simulink model "Battery_detailed_SOC_estimation"  (R2023b)
settings: Solver=VariableStepAuto  StartTime=0.0  StopTime=6*3600  RelTol=1e-3
InitFcn:
  | initialSOC = 0.5;
  | Ts = 1;
libraries: nesl_utility x4, fl_lib x3, simulink x3, batteryecm_lib x1
settings Model: Creator=arvba41  LastModifiedBy=arvba41

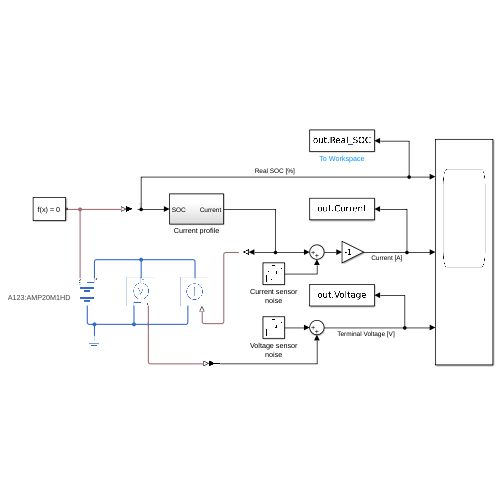
[thumbnail: Simulink's stored preview of the top-level diagram]
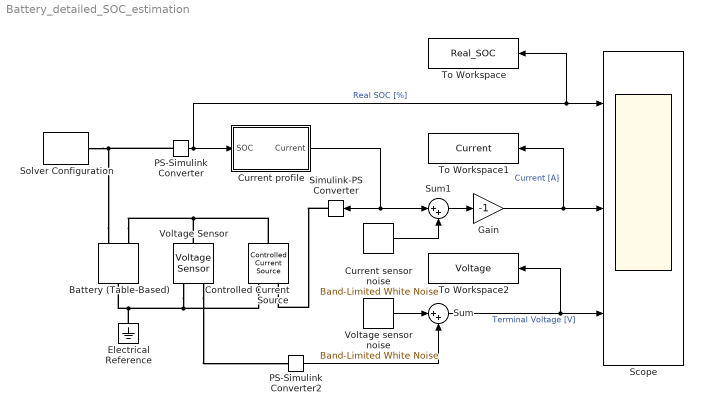
== system Battery_detailed_SOC_estimation ==
  Battery (Table-Based) : batteryecm_lib/Battery (Table-Based)  Tag={'toolbox/physmod/battery/shared_library/m/batteryecm_lib_parts';'Battery__Table_Based_/A123/AMP20M1HD.xml'}  SOC_vec=[0 0.01 0.02 0.03 0.04 0.05 0.06 0.07 0.08 0.09 0.1 0.11 0.12 0.13 0.14 0.15 0.16 0.17 0.18 0.19 0.2 0.21 0.22 0.23 0.24 0.25 0.26 0.27 0.28 0.29 0.3 0.31 0.32 0.33 0.34 0.35 0.36 0.37 0.38 0.39 0.4 0.41 0.42 0.43 0.44 0.45 0.46 0.47 0.48 0.49 0.5 0.51 0.52 0.53 0.54 0.55 0.56 0.57 0.58 0.59 0.6 0.61 0.62 0.63 0.64 0.65 0.66 0.67 0.68 0.69 0.7 0.71 0.72 0.73 0.74 0.75 0.76 0.77 0.78 0.79 0.8 0.81 0.82 0.83 0.84 0.85 0.86 0.87 0.88 0.89 0.9 0.91 0.92 0.93 0.94 0.95 0.96 0.97 0.98 0.99 1]  T_dependence=simscape.enum.tablebattery.temperature_dependence.yes  prm_dir=simscape.enum.tablebattery.prm_dir.noCurrentDirectionality  T_vec=[-10 0 10 25 35] degC  V0_mat=[2.93217 2.93217 2.93217 2.93217 2.93217;2.94263 2.94263 2.94263 2.94263 2.94263;2.95309 2.95309 2.95309 2.95309 2.95309;2.96355 2.96355 2.96355 2.96355 2.96355;2.97401 2.97401 2.97401 2.97401 2.97401;2.98447 2.98447 2.98447 2.98447 2.98447;2.99493 2.99493 2.99493 2.99493 2.99493;3.02455 3.02455 3.02455 3.02455 3.02455;3.05382 3.05382 3.05382 3.05382 3.05382;3.07377 3.07377 3.07377 3.07377 3.07377;3.08453 3.08453 3.08453 3.08453 3.08453;3.09529 3.09529 3.09529 3.09529 3.09529;3.09916 3.09916 3.09916 3.09916 3.09916;3.10271 3.10271 3.10271 3.10271 3.10271;3.10625 3.10625 3.10625 3.10625 3.10625;3.1098 3.1098 3.1098 3.1098 3.1098;3.11335 3.11335 3.11335 3.11335 3.11335;3.11689 3.11689 3.11689 3.11689 3.11689;3.12044 3.12044 3.12044 3.12044 3.12044;3.13089 3.13089 3.13089 3.13089 3.13089;3.13795 3.13795 3.13795 3.13795 3.13795;3.14459 3.14459 3.14459 3.14459 3.14459;3.14961 3.14961 3.14961 3.14961 3.14961;3.15451 3.15451 3.15451 3.15451 3.15451;3.15932 3.15932 3.15932 3.15932 3.15932;3.16324 3.16324 3.16324 3.16324 3.16324;3.16716 3.16716 3.16716 3.16716 3.16716;3.17063 3.17063 3.17063 3.17063 3.17063;3.17297 3.17297 3.17297 3.17297 3.17297;3.17544 3.17544 3.17544 3.17544 3.17544;3.17798 3.17798 3.17798 3.17798 3.17798;3.18052 3.18052 3.18052 3.18052 3.18052;3.18295 3.18295 3.18295 3.18295 3.18295;3.18533 3.18533 3.18533 3.18533 3.18533;3.18771 3.18771 3.18771 3.18771 3.18771;3.19009 3.19009 3.19009 3.19009 3.19009;3.19215 3.19215 3.19215 3.19215 3.19215;3.19403 3.19403 3.19403 3.19403 3.19403;3.1959 3.1959 3.1959 3.1959 3.1959;3.19777 3.19777 3.19777 3.19777 3.19777;3.1998 3.1998 3.1998 3.1998 3.1998;3.20198 3.20198 3.20198 3.20198 3.20198;3.20371 3.20371 3.20371 3.20371 3.20371;3.20501 3.20501 3.20501 3.20501 3.20501;3.20619 3.20619 3.20619 3.20619 3.20619;3.20738 3.20738 3.20738 3.20738 3.20738;3.20856 3.20856 3.20856 3.20856 3.20856;3.20974 3.20974 3.20974 3.20974 3.20974;3.21092 3.21092 3.21092 3.21092 3.21092;3.2121 3.2121 3.2121 3.2121 3.2121;3.21329 3.21329 3.21329 3.21329 3.21329;3.21447 3.21447 3.21447 3.21447 3.21447;3.21565 3.21565 3.21565 3.21565 3.21565;3.21672 3.21672 3.21672 3.21672 3.21672;3.21787 3.21787 3.21787 3.21787 3.21787;3.21904 3.21904 3.21904 3.21904 3.21904;3.22021 3.22021 3.22021 3.22021 3.22021;3.22139 3.22139 3.22139 3.22139 3.22139;3.22256 3.22256 3.22256 3.22256 3.22256;3.22374 3.22374 3.22374 3.22374 3.22374;3.22492 3.22492 3.22492 3.22492 3.22492;3.2261 3.2261 3.2261 3.2261 3.2261;3.22728 3.22728 3.22728 3.22728 3.22728;3.22847 3.22847 3.22847 3.22847 3.22847;3.22965 3.22965 3.22965 3.22965 3.22965;3.23083 3.23083 3.23083 3.23083 3.23083;3.23201 3.23201 3.23201 3.23201 3.23201;3.23319 3.23319 3.23319 3.23319 3.23319;3.23437 3.23437 3.23437 3.23437 3.23437;3.23552 3.23552 3.23552 3.23552 3.23552;3.23652 3.23652 3.23652 3.23652 3.23652;3.23778 3.23778 3.23778 3.23778 3.23778;3.23909 3.23909 3.23909 3.23909 3.23909;3.24045 3.24045 3.24045 3.24045 3.24045;3.24217 3.24217 3.24217 3.24217 3.24217;3.2439 3.2439 3.2439 3.2439 3.2439;3.24563 3.24563 3.24563 3.24563 3.24563;3.24736 3.24736 3.24736 3.24736 3.24736;3.24909 3.24909 3.24909 3.24909 3.24909;3.25082 3.25082 3.25082 3.25082 3.25082;3.25255 3.25255 3.25255 3.25255 3.25255;3.25428 3.25428 3.25428 3.25428 3.25428;3.256 3.256 3.256 3.256 3.256;3.25774 3.25774 3.25774 3.25774 3.25774;3.25951 3.25951 3.25951 3.25951 3.25951;3.26116 3.26116 3.26116 3.26116 3.26116;3.26238 3.26238 3.26238 3.26238 3.26238;3.26307 3.26307 3.26307 3.26307 3.26307;3.26352 3.26352 3.26352 3.26352 3.26352;3.26396 3.26396 3.26396 3.26396 3.26396;3.26441 3.26441 3.26441 3.26441 3.26441;3.26485 3.26485 3.26485 3.26485 3.26485;3.2653 3.2653 3.2653 3.2653 3.2653;3.26593 3.26593 3.26593 3.26593 3.26593;3.26612 3.26612 3.26612 3.26612 3.26612;3.26743 3.26743 3.26743 3.26743 3.26743;3.26879 3.26879 3.26879 3.26879 3.26879;3.27596 3.27596 3.27596 3.27596 3.27596;3.2842 3.2842 3.2842 3.2842 3.2842;3.30299 3.30299 3.30299 3.30299 3.30299;3.33677 3.33677 3.33677 3.33677 3.33677] V  V0_vec=[2.93217 2.94263 2.95309 2.96355 2.97401 2.98447 2.99493 3.02455 3.05382 3.07377 3.08453 3.09529 3.09916 3.10271 3.10625 3.1098 3.11335 3.11689 3.12044 3.13089 3.13795 3.14459 3.14961 3.15451 3.15932 3.16324 3.16716 3.17063 3.17297 3.17544 3.17798 3.18052 3.18295 3.18533 3.18771 3.19009 3.19215 3.19403 3.1959 3.19777 3.1998 3.20198 3.20371 3.20501 3.20619 3.20738 3.20856 3.20974 3.21092 3.2121 3.21329 3.21447 3.21565 3.21672 3.21787 3.21904 3.22021 3.22139 3.22256 3.22374 3.22492 3.2261 3.22728 3.22847 3.22965 3.23083 3.23201 3.23319 3.23437 3.23552 3.23652 3.23778 3.23909 3.24045 3.24217 3.2439 3.24563 3.24736 3.24909 3.25082 3.25255 3.25428 3.256 3.25774 3.25951 3.26116 3.26238 3.26307 3.26352 3.26396 3.26441 3.26485 3.2653 3.26593 3.26612 3.26743 3.26879 3.27596 3.2842 3.30299 3.33677] V  V_range=[1.8 Inf] V  R0_mat=[0.07996 0.07435 0.07218 0.00349 0.04758;0.07879 0.07234 0.06844 0.0033 0.01888;0.07763 0.07033 0.0647 0.00311 0.01407;0.07646 0.06833 0.06096 0.00292 0.00948;0.07529 0.06632 0.05722 0.00272 0.0049;0.07413 0.06432 0.05347 0.00253 0.00119;0.07296 0.06231 0.04973 0.00235 0.00022;0.07278 0.06129 0.04698 0.00233 0.00024;0.07258 0.06024 0.0446 0.00235 0.00024;0.0719 0.05873 0.04247 0.00232 0.00024;0.07075 0.05673 0.03988 0.00223 0.00024;0.0696 0.05474 0.03743 0.00214 0.00024;0.06809 0.0524 0.03472 0.00205 0.00024;0.06657 0.05004 0.032 0.00196 0.00024;0.06505 0.04768 0.02927 0.00187 0.00024;0.06353 0.04532 0.02655 0.00181 0.00024;0.06201 0.04298 0.02426 0.00175 0.00024;0.06049 0.04073 0.02215 0.00169 0.00024;0.05897 0.03848 0.02004 0.00164 0.00024;0.0578 0.03658 0.01828 0.00167 0.0006;0.05646 0.03451 0.01635 0.00168 0.00078;0.0551 0.03261 0.01479 0.00168 0.00094;0.05366 0.03068 0.01317 0.00168 0.00101;0.0522 0.02875 0.01154 0.00168 0.00108;0.05075 0.02681 0.01054 0.00167 0.00114;0.04925 0.02502 0.01001 0.00167 0.00116;0.04759 0.02356 0.00948 0.00167 0.00118;0.04591 0.02208 0.00893 0.00167 0.00118;0.04416 0.02054 0.00832 0.00166 0.00112;0.04243 0.01901 0.00772 0.00165 0.00111;0.0407 0.01812 0.00742 0.00164 0.00113;0.03899 0.01727 0.0072 0.00164 0.00115;0.03731 0.01641 0.00697 0.00163 0.00116;0.03563 0.01555 0.00675 0.00163 0.00117;0.03395 0.01474 0.00652 0.00162 0.00119;0.03227 0.01421 0.0063 0.00162 0.0012;0.03067 0.01366 0.00605 0.00161 0.00119;0.02945 0.0131 0.00583 0.0016 0.00118;0.02823 0.01254 0.0058 0.00159 0.00117;0.02701 0.01213 0.00577 0.00159 0.00115;0.02586 0.01192 0.00574 0.00158 0.00115;0.02512 0.01173 0.00573 0.00158 0.00115;0.02436 0.01151 0.00569 0.00158 0.00113;0.02358 0.01127 0.00563 0.00157 0.00109;0.02279 0.01107 0.00557 0.00156 0.00111;0.022 0.01096 0.0055 0.00156 0.00112;0.02121 0.01085 0.00544 0.00155 0.00114;0.02046 0.01074 0.00537 0.00154 0.00115;0.0201 0.01063 0.00534 0.00154 0.00117;0.01974 0.01052 0.00531 0.00153 0.00118;0.01938 0.01042 0.00528 0.00153 0.00119;0.01902 0.01031 0.00526 0.00152 0.00121;0.01865 0.0102 0.00523 0.00151 0.00122;0.01829 0.01009 0.00519 0.00151 0.00123;0.01792 0.00998 0.00516 0.0015 0.00124;0.01756 0.00987 0.00513 0.0015 0.00126;0.01735 0.00976 0.0051 0.0015 0.00127;0.01723 0.00967 0.00507 0.00149 0.00128;0.01712 0.00965 0.00504 0.00149 0.0013;0.017 0.00963 0.00501 0.00149 0.00131;0.01688 0.00961 0.00498 0.00148 0.00133;0.01676 0.00959 0.00496 0.00148 0.00134;0.01665 0.00957 0.00493 0.00148 0.00135;0.01653 0.00955 0.0049 0.00147 0.00137;0.01641 0.00953 0.00488 0.00147 0.00138;0.01629 0.00951 0.00485 0.00147 0.0014;0.01618 0.00949 0.00482 0.00147 0.00141;0.01606 0.00947 0.00479 0.00146 0.00142;0.01594 0.00945 0.00477 0.00146 0.00143;0.01589 0.00942 0.00474 0.00146 0.00141;0.01586 0.00937 0.0047 0.00145 0.00139;0.01584 0.00934 0.00468 0.00146 0.00139;0.01583 0.0093 0.00466 0.00146 0.00138;0.01581 0.00927 0.00464 0.00147 0.00138;0.01582 0.00926 0.00464 0.00147 0.0014;0.01583 0.00925 0.00464 0.00148 0.00141;0.01583 0.00924 0.00465 0.00149 0.00143;0.01584 0.00923 0.00465 0.0015 0.00145;0.01584 0.00921 0.00465 0.0015 0.00146;0.01585 0.00923 0.00465 0.00151 0.00148;0.01585 0.00925 0.00465 0.00152 0.0015;0.01586 0.00926 0.00465 0.00153 0.00152;0.01587 0.00928 0.00465 0.00153 0.00153;0.01587 0.0093 0.00464 0.00154 0.00155;0.01588 0.00932 0.00463 0.00155 0.00157;0.01589 0.00933 0.00462 0.00155 0.00158;0.01587 0.00933 0.00459 0.00156 0.00157;0.01582 0.00929 0.00453 0.00155 0.00154;0.01576 0.00924 0.00446 0.00154 0.00146;0.0157 0.00919 0.00438 0.00153 0.00132;0.01564 0.00915 0.00431 0.00152 0.00118;0.01558 0.0091 0.00424 0.00151 0.00103;0.01552 0.00905 0.00416 0.0015 0.00089;0.01539 0.00891 0.0041 0.00148 0.00076;0.01518 0.00871 0.00401 0.00144 0.00061;0.01502 0.00857 0.00398 0.0014 0.00051;0.01487 0.00844 0.00396 0.00137 0.00041;0.01501 0.0086 0.00385 0.00136 0.00062;0.01436 0.00795 0.00371 0.00131 0.00087;0.01329 0.00785 0.00411 0.00127 0.00126;0.01299 0.00622 0.00111 0.00104 0.00185] Ohm  R0_vec=[0.00349 0.0033 0.00311 0.00292 0.00272 0.00253 0.00235 0.00233 0.00235 0.00232 0.00223 0.00214 0.00205 0.00196 0.00187 0.00181 0.00175 0.00169 0.00164 0.00167 0.00168 0.00168 0.00168 0.00168 0.00167 0.00167 0.00167 0.00167 0.00166 0.00165 0.00164 0.00164 0.00163 0.00163 0.00162 0.00162 0.00161 0.0016 0.00159 0.00159 0.00158 0.00158 0.00158 0.00157 0.00156 0.00156 0.00155 0.00154 0.00154 0.00153 0.00153 0.00152 0.00151 0.00151 0.0015 0.0015 0.0015 0.00149 0.00149 0.00149 0.00148 0.00148 0.00148 0.00147 0.00147 0.00147 0.00147 0.00146 0.00146 0.00146 0.00145 0.00146 0.00146 0.00147 0.00147 0.00148 0.00149 0.0015 0.0015 0.00151 0.00152 0.00153 0.00153 0.00154 0.00155 0.00155 0.00156 0.00155 0.00154 0.00153 0.00152 0.00151 0.0015 0.00148 0.00144 0.0014 0.00137 0.00136 0.00131 0.00127 0.00104] Ohm  R0_dis_mat=[.0117, .0085, .009; .011, .0085, .009; .0114, .0087, .0092; .0107, .0082, .0088; .0107, .0083, .0091; .0113, .0085, .0089; .0116, .0085, .0089] % Parameter not set Ohm  R0_dis_vec=[.0085, .0085, .0087, .0082, .0083, .0085, .0085] % Parameter not set Ohm  R0_ch_mat=[.0117, .0085, .009; .011, .0085, .009; .0114, .0087, .0092; .0107, .0082, .0088; .0107, .0083, .0091; .0113, .0085, .0089; .0116, .0085, .0089] % Parameter not set Ohm  R0_ch_vec=[.0085, .0085, .0087, .0082, .0083, .0085, .0085] % Parameter not set Ohm  AH=19.487 hr*A  prm_leak=simscape.enum.tablebattery.prm_leak.disabled  Rleak_vec=[8000, 7000, 6000] % Parameter not set Ohm  Rleak=7e3 % Parameter not set Ohm  extrapolation_option=simscape.enum.extrapolation.nearest  SOC_port=simscape.enum.tablebattery.enable.yes  prm_dyn=simscape.enum.tablebattery.prm_dyn.off  R1_mat=[.0109, .0029, .0013; .0069, .0024, .0012; .0047, .0026, .0013; .0034, .0016, .001; .0033, .0023, .0014; .0033, .0018, .0011; .0028, .0017, .0011] % Parameter not set Ohm  R1_vec=[.0029, .0024, .0026, .0016, .0023, .0018, .0017] % Parameter not set Ohm  tau1_mat=[20, 36, 39; 31, 45, 39; 109, 105, 61; 36, 29, 26; 59, 77, 67; 40, 33, 29; 25, 39, 33] % Parameter not set s  tau1_vec=[36, 45, 105, 29, 77, 33, 39] % Parameter not set s  R2_mat=[.0109, .0029, .0013; .0069, .0024, .0012; .0047, .0026, .0013; .0034, .0016, .001; .0033, .0023, .0014; .0033, .0018, .0011; .0028, .0017, .0011] % Parameter not set Ohm  R2_vec=[.0029, .0024, .0026, .0016, .0023, .0018, .0017] % Parameter not set Ohm  tau2_mat=[20, 36, 39; 31, 45, 39; 109, 105, 61; 36, 29, 26; 59, 77, 67; 40, 33, 29; 25, 39, 33] % Parameter not set s  tau2_vec=[36, 45, 105, 29, 77, 33, 39] % Parameter not set s  R3_mat=[.0109, .0029, .0013; .0069, .0024, .0012; .0047, .0026, .0013; .0034, .0016, .001; .0033, .0023, .0014; .0033, .0018, .0011; .0028, .0017, .0011] % Parameter not set Ohm  R3_vec=[.0029, .0024, .0026, .0016, .0023, .0018, .0017] % Parameter not set Ohm  tau3_mat=[20, 36, 39; 31, 45, 39; 109, 105, 61; 36, 29, 26; 59, 77, 67; 40, 33, 29; 25, 39, 33] % Parameter not set s  tau3_vec=[36, 45, 105, 29, 77, 33, 39] % Parameter not set s  R4_mat=[.0109, .0029, .0013; .0069, .0024, .0012; .0047, .0026, .0013; .0034, .0016, .001; .0033, .0023, .0014; .0033, .0018, .0011; .0028, .0017, .0011] % Parameter not set Ohm  R4_vec=[.0029, .0024, .0026, .0016, .0023, .0018, .0017] % Parameter not set Ohm  tau4_mat=[20, 36, 39; 31, 45, 39; 109, 105, 61; 36, 29, 26; 59, 77, 67; 40, 33, 29; 25, 39, 33] % Parameter not set s  tau4_vec=[36, 45, 105, 29, 77, 33, 39] % Parameter not set s  R5_mat=[.0109, .0029, .0013; .0069, .0024, .0012; .0047, .0026, .0013; .0034, .0016, .001; .0033, .0023, .0014; .0033, .0018, .0011; .0028, .0017, .0011] % Parameter not set Ohm  R5_vec=[.0029, .0024, .0026, .0016, .0023, .0018, .0017] % Parameter not set Ohm  tau5_mat=[20, 36, 39; 31, 45, 39; 109, 105, 61; 36, 29, 26; 59, 77, 67; 40, 33, 29; 25, 39, 33] % Parameter not set s  tau5_vec=[36, 45, 105, 29, 77, 33, 39] % Parameter not set s  prm_fade=simscape.enum.tablebattery.prm_fade.disabled  N0=100 % Parameter not set  dV0=0 % Parameter not set  dR0=0 % Parameter not set  dAH=0 % Parameter not set  dRleak=0 % Parameter not set  dR1=0 % Parameter not set  dR2=0 % Parameter not set  dR3=0 % Parameter not set  dR4=0 % Parameter not set  dR5=0 % Parameter not set  N0vec=[0 66 131 196 261 326 391 456 521 586 651 716 781 846 911 976 1041 1106 1171 1236 1301 1366 1431 1496 1561 1626 1691 1756 1821 1886 1951 2016 2081 2146 2211 2276 2341 2406 2471 2536 2601 2666 2731 2796 2861 2926 2991 3056 3121 3186 3251 3316 3381 3446 3511 3576 3641 3706 3771 3836 3901 3966 4031 4096 4161 4226 4291 4356 4421 4486 4551 4616 4681 4746 4811 4876 4941 5006 5071 5136 5201 5266 5331 5396 5461 5526 5591 5656 5721 5786 5851 5916 5981 6046 6111 6176 6241 6306 6371 6436]  Tfadevec=[298.15, 323.15] % Parameter not set K  dV0vec=[0 -0.3227 -0.6453 -0.9509 -1.1187 -1.2594 -1.4 -1.5407 -1.6219 -1.683 -1.7439 -1.8049 -1.8602 -1.9134 -1.9665 -2.0196 -2.0441 -2.0544 -2.0647 -2.075 -2.085 -2.0949 -2.1048 -2.1146 -2.1183 -2.1198 -2.1212 -2.1226 -2.1259 -2.1303 -2.1347 -2.1391 -2.1431 -2.1462 -2.1493 -2.1524 -2.1556 -2.1591 -2.1625 -2.166 -2.1695 -2.1729 -2.1764 -2.1798 -2.1833 -2.1867 -2.1902 -2.1936 -2.197 -2.2002 -2.2034 -2.2067 -2.2106 -2.2156 -2.2206 -2.2256 -2.2316 -2.2405 -2.2493 -2.2582 -2.2676 -2.2798 -2.292 -2.3042 -2.3164 -2.3294 -2.3424 -2.3556 -2.3688 -2.3818 -2.3947 -2.4077 -2.4207 -2.4336 -2.4465 -2.4594 -2.4722 -2.485 -2.4978 -2.5106 -2.5233 -2.5361 -2.5489 -2.5617 -2.5745 -2.5872 -2.5999 -2.6126 -2.6253 -2.6381 -2.6508 -2.6635 -2.6765 -2.6898 -2.703 -2.7163 -2.7295 -2.7428 -2.756 -2.7693]  dR0vec=[0 0 0 0 0 0 0 0 0 0 0 0 0 0 0 0 0 0 0 0 0 0 0 0 0 0 0 0 0 0 0 0 0 0 0 0 0 0 0 0 0 0 0 0 0 0 0 0 0 0 0 0 0 0 0 0 0 0 0 0 0 0 0 0 0 0 0 0 0 0 0 0 0 0 0 0 0 0 0 0 0 0 0 0 0 0 0 0 0 0 0 0 0 0 0 0 0 0 0 0] % Parameter assumed  dAHvec=[0 -0.319 -0.638 -0.939 -1.189 -1.439 -1.688 -1.938 -2.188 -2.435 -2.682 -2.93 -3.177 -3.424 -3.671 -3.918 -4.169 -4.421 -4.673 -4.925 -5.177 -5.429 -5.681 -5.933 -6.185 -6.437 -6.683 -6.917 -7.152 -7.386 -7.621 -7.855 -8.09 -8.324 -8.558 -8.793 -9.033 -9.292 -9.551 -9.809 -10.068 -10.327 -10.586 -10.845 -11.104 -11.363 -11.622 -11.88 -12.132 -12.374 -12.616 -12.857 -13.099 -13.341 -13.582 -13.824 -14.066 -14.307 -14.549 -14.791 -15.035 -15.281 -15.526 -15.772 -16.017 -16.263 -16.508 -16.757 -17.007 -17.256 -17.506 -17.755 -18.005 -18.254 -18.504 -18.752 -18.999 -19.246 -19.493 -19.74 -19.986 -20.233 -20.48 -20.727 -20.973 -21.219 -21.464 -21.71 -21.955 -22.201 -22.446 -22.692 -22.943 -23.199 -23.455 -23.711 -23.966 -24.222 -24.478 -24.733]  dRleakvec=[0, 0, 0] % Parameter not set  dR1vec=[0, 0, 0] % Parameter not set  dR2vec=[0, 0, 0] % Parameter not set  dR3vec=[0, 0, 0] % Parameter not set  dR4vec=[0, 0, 0] % Parameter not set  dR5vec=[0, 0, 0] % Parameter not set  dV0mat=[0, 0; 0, 0; 0, 0] % Parameter not set  dR0mat=[0, 0; 0, 0; 0, 0] % Parameter not set  dAHmat=[0, 0; 0, 0; 0, 0] % Parameter not set  dRleakmat=[0, 0; 0, 0; 0, 0] % Parameter not set  dR1mat=[0, 0; 0, 0; 0, 0] % Parameter not set  dR2mat=[0, 0; 0, 0; 0, 0] % Parameter not set  dR3mat=[0, 0; 0, 0; 0, 0] % Parameter not set  dR4mat=[0, 0; 0, 0; 0, 0] % Parameter not set  dR5mat=[0, 0; 0, 0; 0, 0] % Parameter not set  prm_age_modeling=simscape.enum.tablebattery.prm_age_modeling.equation  storage_dt_age_vec=[0] % Parameter not set d  storage_T_age_vec=[273] % Parameter not set K  prm_age_OCV=simscape.enum.tablebattery.prm_age_OCV.OCV  OCV_age=0.9 % Parameter not set  SOC_age=0.6 % Parameter not set  prm_age_resistance=simscape.enum.tablebattery.prm_age.disabled  OCV_scaling_age_resistance=2.2134e6 % Parameter not set  OCV_offset_age_resistance=1.632e6 % Parameter not set  temp_exp_age_resistance=0.515833569 % Parameter not set V  t_exp_age_resistance=0.75 % Parameter not set  T_age_vec_resistance=[273.15, 298.15, 323.15] % Parameter not set K  dt_age_vec_resistance=[90, 180, 270, 360] % Parameter not set d  dR0_age_vec=[0, 0, 0] % Parameter not set  t_meas_dR0_age=100 % Parameter not set d  dR0_age_mat=[0, 0, 0; 0, 0, 0; 0, 0, 0; 0, 0, 0] % Parameter not set  prm_age_capacity=simscape.enum.tablebattery.prm_age.disabled  OCV_scaling_age_capacity=1.5097e07 % Parameter not set  OCV_offset_age_capacity=8.3625e06 % Parameter not set  temp_exp_age_capacity=0.6011 % Parameter not set V  t_exp_age_capacity=0.75 % Parameter not set  T_age_vec_capacity=[273.15, 298.15, 323.15] % Parameter not set K  dt_age_vec_capacity=[90, 180, 270, 360] % Parameter not set d  dAH_age_vec=[0, 0, 0] % Parameter not set  t_meas_dAH_age=100 % Parameter not set d  dAH_age_mat=[0, 0, 0; 0, 0, 0; 0, 0, 0; 0, 0, 0] % Parameter not set  thermal_port=simscape.enum.thermaleffects.omit  temperature=298.15 % Parameter not set K  thermal_mass=446.4 % Parameter assumed J/K  i_specify=off  i_priority=None  i=0 A  i_nominal_specify=off  i_nominal_unit=A  i_nominal_value=1  v_specify=off  v_priority=None  v=0 V  v_nominal_specify=off  v_nominal_unit=V  v_nominal_value=1  stateOfCharge_specify=on  stateOfCharge_priority=High  stateOfCharge=initialSOC  stateOfCharge_nominal_specify=off  stateOfCharge_nominal_unit=1  stateOfCharge_nominal_value=1  num_cycles_specify=off  num_cycles_priority=High  num_cycles=0  num_cycles_nominal_specify=off  num_cycles_nominal_unit=1  num_cycles_nominal_value=1  cell_temperature_specify=off  cell_temperature_priority=High  cell_temperature=293.15 K  cell_temperature_nominal_specify=off  cell_temperature_nominal_unit=K  cell_temperature_nominal_value=1
      settings: AttributesFormatString=A123:AMP20M1HD  InternalSimscapePortConfiguration="{\"Bottom\":[],\"Left\":[{\"id\":\"p\",\"label\":\"+\",\"type\":\"foundation.electrical.electrical\"},{\"id\":\"soc\",\"label\":\"SOC\",\"type\":\"output\"}],\"Right\":[{\"id\":\"n\",\"label\":\"-\",\"type\":\"foundation.electrical.electrical\"}],\"Top\":[]}"
  Controlled Current Source : fl_lib/Electrical/Electrical Sources/Controlled Current Source
  Current profile : Subsystem
  Current sensor noise : simulink/Sources/Band-Limited White Noise  Cov=1e-2  Ts=1  seed=1234
  Electrical Reference : fl_lib/Electrical/Electrical Elements/Electrical Reference
  Gain : Gain  Gain=-1
  PS-Simulink Converter : nesl_utility/PS-Simulink Converter  PhysicalDomain=network_engine_domain  SubClassName=ps_output  LeftPortType=input  RightPortType=output  PseudoPeriodic=off  Frequencies=[]  VectorFormat=inherit  Unit=inherit  AffineConversion=off
  PS-Simulink Converter2 : nesl_utility/PS-Simulink Converter  PhysicalDomain=network_engine_domain  SubClassName=ps_output  LeftPortType=input  RightPortType=output  PseudoPeriodic=off  Frequencies=[]  VectorFormat=inherit  Unit=inherit  AffineConversion=off
  Scope : Scope  NumInputPorts=3
  Simulink-PS Converter : nesl_utility/Simulink-PS Converter  PhysicalDomain=network_engine_domain  SubClassName=ps_input  LeftPortType=input  RightPortType=output  PseudoPeriodic=off  Frequencies=[]  NoiseDistribution=none  NoiseParameters=[]  Unit=1  AffineConversion=off  FilteringAndDerivatives=provide  SimscapeFilterOrder=1  InputFilterTimeConstant=0.001  UdotUserProvided=0
  Solver Configuration : nesl_utility/Solver Configuration  PhysicalDomain=network_engine_domain  SubClassName=solver  LeftPortType=input  RightPortType=generic  Tones=[]  Harmonics=[]  SimulateNoise=off  Profile=off  UseLocalSampling=off  EnableSwitchedLinearOptims=on  FrequencyDomain=off  UseCCode=off  RelTol=0.001  AbsTol=0.001  MinStep=1e-09  ToWorkspace=off  RevertToSquareIcSolve=off  NumHomotopyIterations=100  PhasorMode=off  PhasorModeNumHarmonics=1  ConsistencySolver=NEWTON_XTOL_AFTER_FTOL  IndexReductionMethod=DerivativeReplacement  DoDC=off  ResidualTolerance=1e-09  ConsistencyTolSource=GLOBAL  ConsistencyAbsTol=0.001  ConsistencyRelTol=0.001  ConsistencyTolFactor=0.001  UseLocalSolver=on  LocalSolverChoice=NE_BACKWARD_EULER_ADVANCER  ResolveIndetEquations=on  FunctionEvalNumThread=1  LocalSolverSampleTime=1  DoFixedCost=on  MaxNonlinIter=3  MaxModeIter=2  ComputeImpulses=off  ImpulseIterations=2  LinearAlgebra=auto  LinearAlgebraNumThread=0  EquationFormulation=NE_TIME_EF  DelaysMemoryBudget=1024  AutomaticFiltering=on  FilteringTimeConstant=0.001  PartitionStorageMethod=AS_NEEDED  PartitionMemoryBudget=1024  PartitionMethod=ROBUST  MultibodyUseLocalSolver=off  MultibodyLocalSolverChoice=ODE1  MultibodyLocalSolverSampleTime=0.001
  Sum : Sum  Inputs=|++
  Sum1 : Sum  Inputs=|++
  To Workspace : ToWorkspace  VariableName=Real_SOC  SampleTime=-1
      settings: Save2DSignal=2-D array (concatenate along first dimension)
  To Workspace1 : ToWorkspace  VariableName=Current  SampleTime=-1
      settings: Save2DSignal=2-D array (concatenate along first dimension)
  To Workspace2 : ToWorkspace  VariableName=Voltage  SampleTime=-1
      settings: Save2DSignal=2-D array (concatenate along first dimension)
  Voltage Sensor : fl_lib/Electrical/Electrical Sensors/Voltage Sensor
  Voltage sensor noise : simulink/Sources/Band-Limited White Noise  Cov=1e-3  Ts=1  seed=1234
  wires:
  Voltage sensor noise/1 -> Sum/1
  PS-Simulink Converter2/1 -> Sum/2
  PS-Simulink Converter/1 -> To Workspace/1, Scope/1, Current profile/1(SOC)  "Real SOC [%]"
  Sum1/1 -> Gain/1
  Current sensor noise/1 -> Sum1/2
  Sum/1 -> To Workspace2/1, Scope/3  "Terminal Voltage [V]"
  Current profile/1(Current) -> Sum1/1, Simulink-PS Converter/1
  Gain/1 -> To Workspace1/1, Scope/2  "Current [A]"
  connections:
  Battery (Table-Based)/RConn1 -- Electrical Reference/LConn1 -- Voltage Sensor/RConn2 -- Controlled Current Source/RConn2
  Battery (Table-Based)/LConn1 -- Voltage Sensor/LConn1 -- Controlled Current Source/LConn1
  Battery (Table-Based)/LConn2 -- PS-Simulink Converter/LConn1 -- Solver Configuration/RConn1
  Voltage Sensor/RConn1 -- PS-Simulink Converter2/LConn1
  Simulink-PS Converter/RConn1 -- Controlled Current Source/RConn1

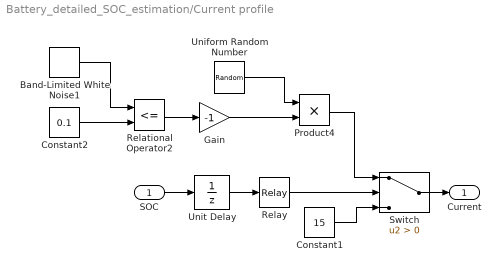
== system Battery_detailed_SOC_estimation/Current profile ==
  SOC : Inport
  Band-Limited White Noise1 : simulink/Sources/Band-Limited White Noise  Cov=1  Ts=50  seed=[23341]
  Constant1 : Constant  Value=15
  Constant2 : Constant  Value=0.1
  Gain : Gain  Gain=-1
  Product4 : Product
  Relational Operator2 : RelationalOperator  Operator=<=  OutDataTypeStr=boolean  RndMeth=Simplest  InputSameDT=off
  Relay : Relay  OnSwitchValue=0.9  OffSwitchValue=0.3  OffOutputValue=-1
  Switch : Switch  Criteria=u2 > Threshold  SaturateOnIntegerOverflow=off  InputSameDT=off
  Uniform Random Number : UniformRandomNumber  Minimum=5  Maximum=55  SampleTime=100
  Unit Delay : UnitDelay  InitialCondition=Ts  SampleTime=Ts  HasFrameUpgradeWarning=on
  Current : Outport
  wires:
  SOC/1 -> Unit Delay/1
  Constant1/1 -> Switch/3
  Relay/1 -> Switch/2
  Product4/1 -> Switch/1
  Unit Delay/1 -> Relay/1
  Switch/1 -> Current/1
  Uniform Random Number/1 -> Product4/1
  Band-Limited White Noise1/1 -> Relational Operator2/1
  Gain/1 -> Product4/2
  Relational Operator2/1 -> Gain/1
  Constant2/1 -> Relational Operator2/2
